simulink model "panModelPredictiveControl2012"  (R2021a)
settings: Solver=FixedStepAuto  StartTime=0.0  StopTime=10  FixedStep=0.01  RelTol=1e-3
settings Model: Creator=randolf  LastModifiedBy=randolf

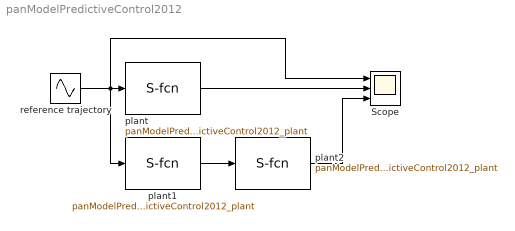
== system panModelPredictiveControl2012 ==
  Scope : Scope  NumInputPorts=3
  plant : M-S-Function  FunctionName=panModelPredictiveControl2012_plant  Parameters=[1,0,0],[0, 0]
  plant1 : M-S-Function  FunctionName=panModelPredictiveControl2012_plant  Parameters=[1,0,0],[0, 0]
  plant2 : M-S-Function  FunctionName=panModelPredictiveControl2012_plant  Parameters=[1,0,0],[0, 0]
  reference trajectory : Sin  SampleTime=0
  wires:
  plant/1 -> Scope/2
  reference trajectory/1 -> Scope/1, plant/1, plant1/1
  plant1/1 -> plant2/1
  plant2/1 -> Scope/3
